simulink model "Problem4"  (R2020a)
settings: Solver=VariableStepAuto  StartTime=0.0  StopTime=10.0  RelTol=1e-3
settings Model: Creator=kasutav  LastModifiedBy=kasutav

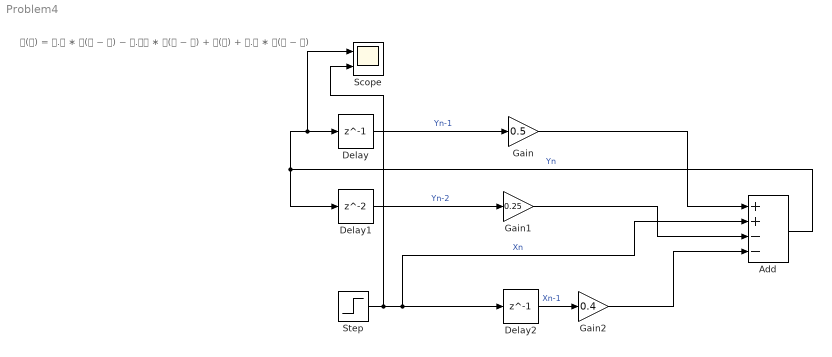
== system Problem4 ==
  note: 𝐲(𝐧) = 𝟎.𝟓 ∗ 𝐲(𝐧 − 𝟏) − 𝟎.𝟐𝟓 ∗ 𝐲(𝐧 − 𝟐) + 𝐱(𝐧) + 𝟎.𝟒 ∗ 𝐱(𝐧 − 𝟏)
  Add : Sum  Inputs=++--
  Delay : Delay  DelayLength=1
  Delay1 : Delay
  Delay2 : Delay  DelayLength=1
  Gain : Gain  Gain=0.5
  Gain1 : Gain  Gain=0.25
  Gain2 : Gain  Gain=0.4
  Scope : Scope  NumInputPorts=2
  Step : Step  SampleTime=0
  wires:
  Add/1 -> Scope/1, Delay/1, Delay1/1  "Yn"
  Delay/1 -> Gain/1  "Yn-1"
  Delay1/1 -> Gain1/1  "Yn-2"
  Step/1 -> Scope/2, Add/2, Delay2/1  "Xn"
  Gain/1 -> Add/1
  Gain1/1 -> Add/3
  Delay2/1 -> Gain2/1  "Xn-1"
  Gain2/1 -> Add/4
